simulink model "Adaptive1dof"  (R2020b)
settings: Solver=VariableStepAuto  StartTime=0.0  StopTime=5  RelTol=1e-3
values from neighbouring files (symbols this model uses):
  K = 0.2    [params.m]
  Kd = diag([0.2])    [params.m]
  lambda = 0.3    [params.m]
libraries: robotcorelib x1
settings Model: Creator=andre  LastModifiedBy=filippo

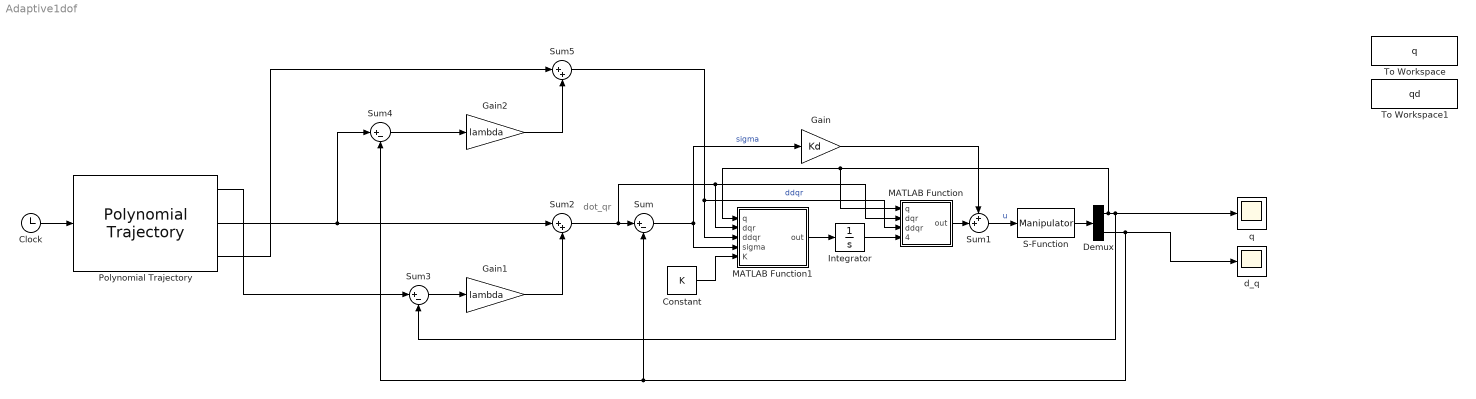
== system Adaptive1dof ==
  note: dot_qr
  Clock : Clock
  Constant : Constant  Value=K
  Demux : Demux  Outputs=2
  Gain : Gain  Gain=Kd
  Gain1 : Gain  Gain=lambda
  Gain2 : Gain  Gain=lambda
  Integrator : Integrator
  MATLAB Function : MATLAB Function  TreatAsAtomicUnit=on
  MATLAB Function1 : MATLAB Function  TreatAsAtomicUnit=on
  Polynomial Trajectory : robotcorelib/Polynomial Trajectory  WaypointSource=Internal  Waypoints=[ 0, 2, 1, 5, 0]  TimePoints=[ 0, 1, 2, 3, 4 ]  TimeInterval=[ 1, 4 ]  Method=Cubic Polynomial  ParameterSource=Internal  VelocityBoundaryCondition=zeros( 1, 5)  AccelerationBoundaryCondition=zeros( 2, 5 )  SimulateUsing=Interpreted execution
  S-Function : S-Function  FunctionName=Manipulator  Parameters=param  SFunctionDeploymentMode=off  EnableBusSupport=off
  Sum : Sum  Inputs=|+-
  Sum1 : Sum  Inputs=++|
  Sum2 : Sum  Inputs=|++
  Sum3 : Sum  Inputs=|+-
  Sum4 : Sum  Inputs=|+-
  Sum5 : Sum  Inputs=|++
  To Workspace : ToWorkspace  VariableName=q  SaveFormat=Timeseries  SampleTime=-1
  To Workspace1 : ToWorkspace  VariableName=qd  SaveFormat=Timeseries  SampleTime=-1
  d_q : Scope
  q : Scope
  wires:
  Sum2/1 -> MATLAB Function1/2(dqr), MATLAB Function/2(dqr), Sum/1
  S-Function/1 -> Demux/1
  Sum1/1 -> S-Function/1  "u"
  Demux/1 -> Sum3/2, q/1, MATLAB Function1/1(q), MATLAB Function/1(q)
  Demux/2 -> Sum4/2, Sum/2, d_q/1
  Integrator/1 -> MATLAB Function/4(theta_hat)
  MATLAB Function/1(out) -> Sum1/2
  Sum/1 -> MATLAB Function1/4(sigma), Gain/1  "sigma"
  Gain/1 -> Sum1/1
  Gain1/1 -> Sum2/2
  Sum3/1 -> Gain1/1
  Sum4/1 -> Gain2/1
  Polynomial Trajectory/3 -> Sum5/1
  Gain2/1 -> Sum5/2
  Polynomial Trajectory/2 -> Sum2/1, Sum4/1
  Polynomial Trajectory/1 -> Sum3/1
  Clock/1 -> Polynomial Trajectory/1
  Sum5/1 -> MATLAB Function1/3(ddqr), MATLAB Function/3(ddqr)  "ddqr"
  Constant/1 -> MATLAB Function1/5(K)
  MATLAB Function1/1(out) -> Integrator/1

== matlab function Adaptive1dof/MATLAB Function1 ==
  data: q input; dqr input; out output; ddqr input; sigma input; K input
function out = KY(q,  dqr, ddqr, sigma, K)
    Y = [ddqr, dqr sin(q)];
    
    out = inv(K)*Y'*sigma;
end

== matlab function Adaptive1dof/MATLAB Function ==
  data: q input; dqr input; ddqr input; theta_hat input; out output
function out = Y(q,dqr,ddqr, theta_hat)
    Y = [ddqr, dqr sin(q)];
    
    out = Y*theta_hat;
end
